simulink model "weather_station_system_composer"  (R2019b)
settings: Solver=VariableStepAuto  StartTime=0.0  StopTime=10.0  RelTol=1e-3
settings Model: Creator=Agnieszka  LastModifiedBy=Agnieszka

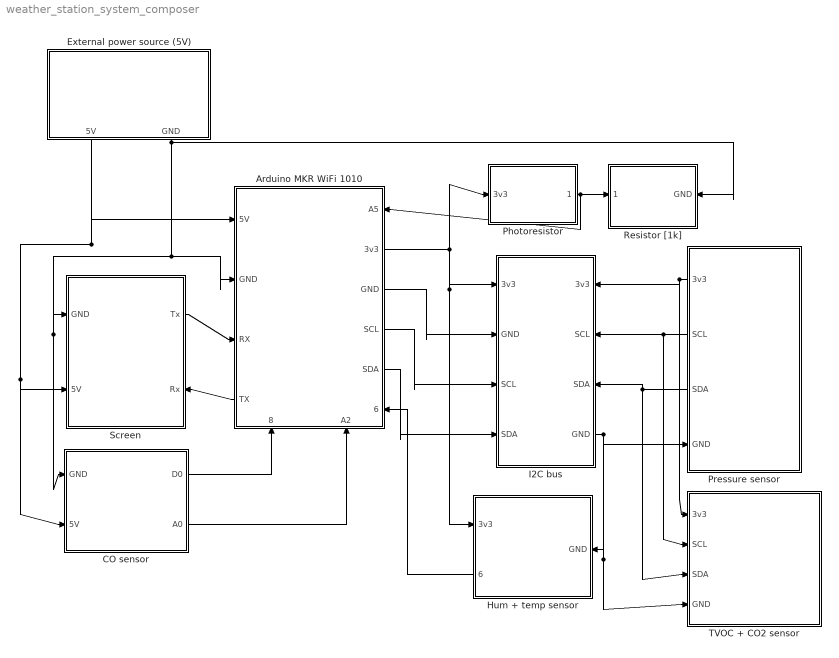
== system weather_station_system_composer ==
  Arduino MKR WiFi 1010 : Subsystem
      settings: PortSchema="{\"entries\":[{\"content\":{\"headerSize\":26,\"margin\":15,\"minimumSpacing\":25,\"sides\":[{\"content\":{\"connectorIds\":[\"In5\",\"In6\",\"In7\",\"Out5\"]},\"type\":\"ConnectorPlacement.EquallySpacedRectSide\",\"uuid\":\"d8843e03-410a-4015-bef5-a60d478fb572\"},{\"content\":{\"connectorIds\":[\"In3\",\"Out1\",\"Out2\",\"Out3\",\"Out4\",\"In4\"],\"side\":\"RIGHT\"},\"type\":\"ConnectorPlacement.EquallySpacedRectSide\",\"uuid\":\"d54f0a32-9d75-4682-a90c-bbeb8f935ea1\"},{\"content\":{\"connectorIds\":[],\"side\":\"TOP\"},\"type\":\"ConnectorPlacement.EquallySpacedRectSide\",\"uuid\":\"edd4fcda-a5fc-4f5e-9afd-4cf040840e08\"},{\"content\":{\"connectorIds\":[\"In1\",\"In2\"],\"side\":\"BOTTOM\"},\"type\":\"ConnectorPlacement.EquallySpacedRectSide\",\"uuid\":\"08268377-cd46-4d21-8d8a-4c68f476b1a8\"}]},\"type\":\"ConnectorPlacement.EquallySpacedConnector\",\"uuid\":\"864dd0c4-ce7b-459e-945c-e91ac4f825e1\"}],\"packageUris\":[\"http://schema.mathworks.com/mf0/Connector/19700101\"],\"version\":\"1.0\"}"
  CO sensor : Subsystem
      settings: PortSchema="{\"entries\":[{\"content\":{\"headerSize\":26,\"margin\":15,\"minimumSpacing\":25,\"sides\":[{\"content\":{\"connectorIds\":[\"In1\",\"In2\"]},\"type\":\"ConnectorPlacement.EquallySpacedRectSide\",\"uuid\":\"d8843e03-410a-4015-bef5-a60d478fb572\"},{\"content\":{\"connectorIds\":[\"Out1\",\"Out2\"],\"side\":\"RIGHT\"},\"type\":\"ConnectorPlacement.EquallySpacedRectSide\",\"uuid\":\"d54f0a32-9d75-4682-a90c-bbeb8f935ea1\"},{\"content\":{\"connectorIds\":[],\"side\":\"TOP\"},\"type\":\"ConnectorPlacement.EquallySpacedRectSide\",\"uuid\":\"edd4fcda-a5fc-4f5e-9afd-4cf040840e08\"}]},\"type\":\"ConnectorPlacement.EquallySpacedConnector\",\"uuid\":\"864dd0c4-ce7b-459e-945c-e91ac4f825e1\"}],\"packageUris\":[\"http://schema.mathworks.com/mf0/Connector/19700101\"],\"version\":\"1.0\"}"
  External power source (5V) : Subsystem
      settings: PortSchema="{\"entries\":[{\"content\":{\"headerSize\":26,\"margin\":15,\"minimumSpacing\":25,\"sides\":[{\"content\":{\"connectorIds\":[]},\"type\":\"ConnectorPlacement.EquallySpacedRectSide\",\"uuid\":\"d8843e03-410a-4015-bef5-a60d478fb572\"},{\"content\":{\"connectorIds\":[],\"side\":\"RIGHT\"},\"type\":\"ConnectorPlacement.EquallySpacedRectSide\",\"uuid\":\"d54f0a32-9d75-4682-a90c-bbeb8f935ea1\"},{\"content\":{\"connectorIds\":[],\"side\":\"TOP\"},\"type\":\"ConnectorPlacement.EquallySpacedRectSide\",\"uuid\":\"edd4fcda-a5fc-4f5e-9afd-4cf040840e08\"},{\"content\":{\"connectorIds\":[\"Out1\",\"Out2\"],\"side\":\"BOTTOM\"},\"type\":\"ConnectorPlacement.EquallySpacedRectSide\",\"uuid\":\"68150884-f07c-4eb8-a887-f336eeb0641e\"}]},\"type\":\"ConnectorPlacement.EquallySpacedConnector\",\"uuid\":\"864dd0c4-ce7b-459e-945c-e91ac4f825e1\"}],\"packageUris\":[\"http://schema.mathworks.com/mf0/Connector/19700101\"],\"version\":\"1.0\"}"
  Hum + temp sensor : Subsystem
      settings: PortSchema="{\"entries\":[{\"content\":{\"headerSize\":26,\"margin\":15,\"minimumSpacing\":25,\"sides\":[{\"content\":{\"connectorIds\":[\"In2\",\"Out1\"]},\"type\":\"ConnectorPlacement.EquallySpacedRectSide\",\"uuid\":\"d8843e03-410a-4015-bef5-a60d478fb572\"},{\"content\":{\"connectorIds\":[\"In1\"],\"side\":\"RIGHT\"},\"type\":\"ConnectorPlacement.EquallySpacedRectSide\",\"uuid\":\"d54f0a32-9d75-4682-a90c-bbeb8f935ea1\"},{\"content\":{\"connectorIds\":[],\"side\":\"TOP\"},\"type\":\"ConnectorPlacement.EquallySpacedRectSide\",\"uuid\":\"edd4fcda-a5fc-4f5e-9afd-4cf040840e08\"}]},\"type\":\"ConnectorPlacement.EquallySpacedConnector\",\"uuid\":\"864dd0c4-ce7b-459e-945c-e91ac4f825e1\"}],\"packageUris\":[\"http://schema.mathworks.com/mf0/Connector/19700101\"],\"version\":\"1.0\"}"
  I2C bus : Subsystem
      settings: PortSchema="{\"entries\":[{\"content\":{\"headerSize\":26,\"margin\":15,\"minimumSpacing\":25,\"sides\":[{\"content\":{\"connectorIds\":[\"In5\",\"In2\",\"In6\",\"In7\"]},\"type\":\"ConnectorPlacement.EquallySpacedRectSide\",\"uuid\":\"d8843e03-410a-4015-bef5-a60d478fb572\"},{\"content\":{\"connectorIds\":[\"In1\",\"In3\",\"In4\",\"Out1\"],\"side\":\"RIGHT\"},\"type\":\"ConnectorPlacement.EquallySpacedRectSide\",\"uuid\":\"d54f0a32-9d75-4682-a90c-bbeb8f935ea1\"},{\"content\":{\"connectorIds\":[],\"side\":\"TOP\"},\"type\":\"ConnectorPlacement.EquallySpacedRectSide\",\"uuid\":\"edd4fcda-a5fc-4f5e-9afd-4cf040840e08\"}]},\"type\":\"ConnectorPlacement.EquallySpacedConnector\",\"uuid\":\"864dd0c4-ce7b-459e-945c-e91ac4f825e1\"}],\"packageUris\":[\"http://schema.mathworks.com/mf0/Connector/19700101\"],\"version\":\"1.0\"}"
  Photoresistor : Subsystem
      settings: PortSchema="{\"entries\":[{\"content\":{\"headerSize\":26,\"margin\":15,\"minimumSpacing\":25,\"sides\":[{\"content\":{\"connectorIds\":[\"In1\"]},\"type\":\"ConnectorPlacement.EquallySpacedRectSide\",\"uuid\":\"d8843e03-410a-4015-bef5-a60d478fb572\"},{\"content\":{\"connectorIds\":[\"Out1\"],\"side\":\"RIGHT\"},\"type\":\"ConnectorPlacement.EquallySpacedRectSide\",\"uuid\":\"d54f0a32-9d75-4682-a90c-bbeb8f935ea1\"},{\"content\":{\"connectorIds\":[],\"side\":\"TOP\"},\"type\":\"ConnectorPlacement.EquallySpacedRectSide\",\"uuid\":\"edd4fcda-a5fc-4f5e-9afd-4cf040840e08\"}]},\"type\":\"ConnectorPlacement.EquallySpacedConnector\",\"uuid\":\"864dd0c4-ce7b-459e-945c-e91ac4f825e1\"}],\"packageUris\":[\"http://schema.mathworks.com/mf0/Connector/19700101\"],\"version\":\"1.0\"}"
  Pressure sensor : Subsystem
      settings: PortSchema="{\"entries\":[{\"content\":{\"headerSize\":26,\"margin\":15,\"minimumSpacing\":25,\"sides\":[{\"content\":{\"connectorIds\":[\"Out1\",\"Out2\",\"Out3\",\"In1\"]},\"type\":\"ConnectorPlacement.EquallySpacedRectSide\",\"uuid\":\"d8843e03-410a-4015-bef5-a60d478fb572\"},{\"content\":{\"connectorIds\":[],\"side\":\"RIGHT\"},\"type\":\"ConnectorPlacement.EquallySpacedRectSide\",\"uuid\":\"d54f0a32-9d75-4682-a90c-bbeb8f935ea1\"},{\"content\":{\"connectorIds\":[],\"side\":\"TOP\"},\"type\":\"ConnectorPlacement.EquallySpacedRectSide\",\"uuid\":\"edd4fcda-a5fc-4f5e-9afd-4cf040840e08\"}]},\"type\":\"ConnectorPlacement.EquallySpacedConnector\",\"uuid\":\"864dd0c4-ce7b-459e-945c-e91ac4f825e1\"}],\"packageUris\":[\"http://schema.mathworks.com/mf0/Connector/19700101\"],\"version\":\"1.0\"}"
  Resistor [1k] : Subsystem
      settings: PortSchema="{\"entries\":[{\"content\":{\"headerSize\":26,\"margin\":15,\"minimumSpacing\":25,\"sides\":[{\"content\":{\"connectorIds\":[\"In2\"]},\"type\":\"ConnectorPlacement.EquallySpacedRectSide\",\"uuid\":\"d8843e03-410a-4015-bef5-a60d478fb572\"},{\"content\":{\"connectorIds\":[\"In1\"],\"side\":\"RIGHT\"},\"type\":\"ConnectorPlacement.EquallySpacedRectSide\",\"uuid\":\"d54f0a32-9d75-4682-a90c-bbeb8f935ea1\"},{\"content\":{\"connectorIds\":[],\"side\":\"TOP\"},\"type\":\"ConnectorPlacement.EquallySpacedRectSide\",\"uuid\":\"edd4fcda-a5fc-4f5e-9afd-4cf040840e08\"}]},\"type\":\"ConnectorPlacement.EquallySpacedConnector\",\"uuid\":\"864dd0c4-ce7b-459e-945c-e91ac4f825e1\"}],\"packageUris\":[\"http://schema.mathworks.com/mf0/Connector/19700101\"],\"version\":\"1.0\"}"
  Screen : Subsystem
      settings: PortSchema="{\"entries\":[{\"content\":{\"headerSize\":26,\"margin\":15,\"minimumSpacing\":25,\"sides\":[{\"content\":{\"connectorIds\":[\"In2\",\"In3\"]},\"type\":\"ConnectorPlacement.EquallySpacedRectSide\",\"uuid\":\"d8843e03-410a-4015-bef5-a60d478fb572\"},{\"content\":{\"connectorIds\":[\"Out1\",\"In1\"],\"side\":\"RIGHT\"},\"type\":\"ConnectorPlacement.EquallySpacedRectSide\",\"uuid\":\"d54f0a32-9d75-4682-a90c-bbeb8f935ea1\"},{\"content\":{\"connectorIds\":[],\"side\":\"TOP\"},\"type\":\"ConnectorPlacement.EquallySpacedRectSide\",\"uuid\":\"edd4fcda-a5fc-4f5e-9afd-4cf040840e08\"}]},\"type\":\"ConnectorPlacement.EquallySpacedConnector\",\"uuid\":\"864dd0c4-ce7b-459e-945c-e91ac4f825e1\"}],\"packageUris\":[\"http://schema.mathworks.com/mf0/Connector/19700101\"],\"version\":\"1.0\"}"
  TVOC + CO2 sensor : Subsystem
      settings: PortSchema="{\"entries\":[{\"content\":{\"headerSize\":26,\"margin\":15,\"minimumSpacing\":25,\"sides\":[{\"content\":{\"connectorIds\":[\"In1\",\"In2\",\"In3\",\"In4\"]},\"type\":\"ConnectorPlacement.EquallySpacedRectSide\",\"uuid\":\"d8843e03-410a-4015-bef5-a60d478fb572\"},{\"content\":{\"connectorIds\":[],\"side\":\"RIGHT\"},\"type\":\"ConnectorPlacement.EquallySpacedRectSide\",\"uuid\":\"d54f0a32-9d75-4682-a90c-bbeb8f935ea1\"},{\"content\":{\"connectorIds\":[],\"side\":\"TOP\"},\"type\":\"ConnectorPlacement.EquallySpacedRectSide\",\"uuid\":\"edd4fcda-a5fc-4f5e-9afd-4cf040840e08\"}]},\"type\":\"ConnectorPlacement.EquallySpacedConnector\",\"uuid\":\"864dd0c4-ce7b-459e-945c-e91ac4f825e1\"}],\"packageUris\":[\"http://schema.mathworks.com/mf0/Connector/19700101\"],\"version\":\"1.0\"}"
  wires:
  External power source (5V)/1(5V) -> Arduino MKR WiFi 1010/5(5V), Screen/3(5V), CO sensor/2(5V)
  External power source (5V)/2(GND) -> Screen/2(GND), CO sensor/1(GND), Arduino MKR WiFi 1010/6(GND), Resistor [1k]/1(GND)
  Screen/1(Tx) -> Arduino MKR WiFi 1010/7(RX)
  Arduino MKR WiFi 1010/5(TX) -> Screen/1(Rx)
  Arduino MKR WiFi 1010/1(3v3) -> Hum + temp sensor/2(3v3), I2C bus/5(3v3), Photoresistor/1(3v3)
  Photoresistor/1(1) -> Arduino MKR WiFi 1010/3(A5), Resistor [1k]/2(1)
  Arduino MKR WiFi 1010/3(SCL) -> I2C bus/6(SCL)
  Arduino MKR WiFi 1010/4(SDA) -> I2C bus/7(SDA)
  Pressure sensor/1(" 3v3") -> TVOC + CO2 sensor/1(3v3), I2C bus/1("  3v3")
  Pressure sensor/2(" SCL") -> TVOC + CO2 sensor/2(SCL), I2C bus/3(" SCL")
  Pressure sensor/3(" SDA") -> I2C bus/4(" SDA"), TVOC + CO2 sensor/3(SDA)
  Hum + temp sensor/1(6) -> Arduino MKR WiFi 1010/4(6)
  CO sensor/1(D0) -> Arduino MKR WiFi 1010/1(8)
  CO sensor/2(A0) -> Arduino MKR WiFi 1010/2(A2)
  Arduino MKR WiFi 1010/2("GND ") -> I2C bus/2("GND  ")
  I2C bus/1(GND) -> Pressure sensor/1(GND), Hum + temp sensor/1(GND), TVOC + CO2 sensor/4(GND)

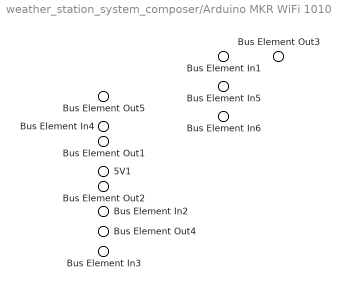
== system weather_station_system_composer/Arduino MKR WiFi 1010 ==
  Bus Element In5 : Inport  PortName=8
  Bus Element In6 : Inport  Port=2  PortName=A2
  Bus Element In1 : Inport  Port=3  PortName=A5
  Bus Element In4 : Inport  Port=4  PortName=6
  5V1 : Inport  Port=5  PortName=5V
  Bus Element In2 : Inport  Port=6  PortName=GND
  Bus Element In3 : Inport  Port=7  PortName=RX
  Bus Element Out3 : Outport  PortName=3v3
  Bus Element Out5 : Outport  Port=2  PortName=GND
  Bus Element Out1 : Outport  Port=3  PortName=SCL
  Bus Element Out4 : Outport  Port=4  PortName=SDA
  Bus Element Out2 : Outport  Port=5  PortName=TX

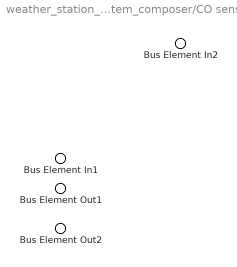
== system weather_station_system_composer/CO sensor ==
  Bus Element In2 : Inport  PortName=GND
  Bus Element In1 : Inport  Port=2  PortName=5V
  Bus Element Out1 : Outport  PortName=D0
  Bus Element Out2 : Outport  Port=2  PortName=A0

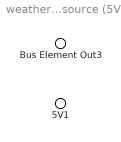
== system weather_station_system_composer/External power source (5V) ==
  5V1 : Outport  PortName=5V
  Bus Element Out3 : Outport  Port=2  PortName=GND

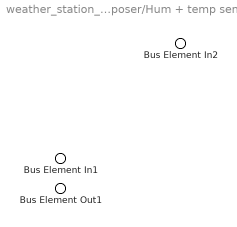
== system weather_station_system_composer/Hum + temp sensor ==
  Bus Element In2 : Inport  PortName=GND
  Bus Element In1 : Inport  Port=2  PortName=3v3
  Bus Element Out1 : Outport  PortName=6

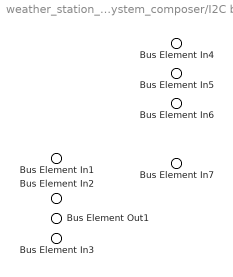
== system weather_station_system_composer/I2C bus ==
  Bus Element In4 : Inport  PortName=3v3
  Bus Element In7 : Inport  Port=2  PortName=GND
  Bus Element In5 : Inport  Port=3  PortName=SCL
  Bus Element In6 : Inport  Port=4  PortName=SDA
  Bus Element In1 : Inport  Port=5  PortName=3v3
  Bus Element In2 : Inport  Port=6  PortName=SCL
  Bus Element In3 : Inport  Port=7  PortName=SDA
  Bus Element Out1 : Outport  PortName=GND

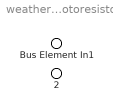
== system weather_station_system_composer/Photoresistor ==
  Bus Element In1 : Inport  PortName=3v3
  2 : Outport  PortName=1

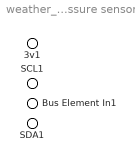
== system weather_station_system_composer/Pressure sensor ==
  Bus Element In1 : Inport  PortName=GND
  " 3v1" : Outport  PortName=3v3
  " SCL1" : Outport  Port=2  PortName=SCL
  " SDA1" : Outport  Port=3  PortName=SDA

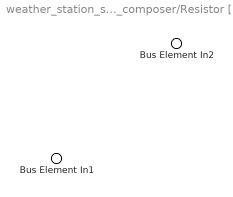
== system weather_station_system_composer/Resistor [1k] ==
  Bus Element In2 : Inport  PortName=GND
  Bus Element In1 : Inport  Port=2  PortName=1

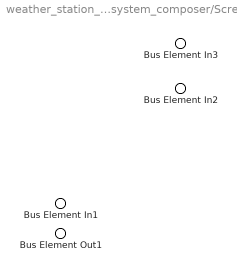
== system weather_station_system_composer/Screen ==
  Bus Element In3 : Inport  PortName=Rx
  Bus Element In2 : Inport  Port=2  PortName=GND
  Bus Element In1 : Inport  Port=3  PortName=5V
  Bus Element Out1 : Outport  PortName=Tx

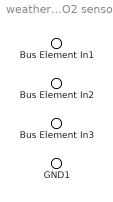
== system weather_station_system_composer/TVOC + CO2 sensor ==
  Bus Element In1 : Inport  PortName=3v3
  Bus Element In2 : Inport  Port=2  PortName=SCL
  Bus Element In3 : Inport  Port=3  PortName=SDA
  GND1 : Inport  Port=4  PortName=GND
